simulink model "KALMAN_2D_test3"  (R2020a)
settings: Solver=VariableStepAuto  StartTime=0.0  StopTime=10  RelTol=1e-3
undefined symbols (not defined in the file): sigbuilder_block
libraries: simulink x3
settings Model: Creator=abdou  LastModifiedBy=abdou

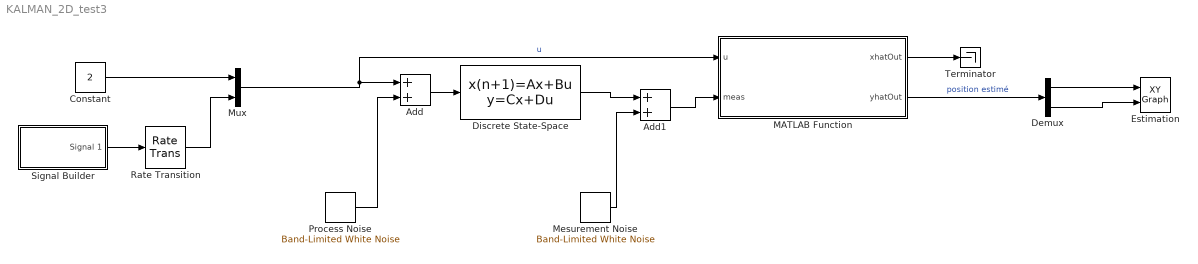
== system KALMAN_2D_test3 ==
  Add : Sum
  Add1 : Sum
  Constant : Constant  Value=2
  Demux : Demux  Outputs=2
  Discrete State-Space : DiscreteStateSpace  A=[1 0; 0 1]  B=[0.1 0; 0 0.1]  C=[1 0; 0 1]  D=[0 0; 0 0]  SampleTime=-1
  Estimation : simulink/Sinks/XY Graph  xmin=0  xmax=20  ymin=-0.2  ymax=0.2  st=-1
  MATLAB Function : MATLAB Function  TreatAsAtomicUnit=on
  Mesurement Noise : simulink/Sources/Band-Limited White Noise  Cov=[1 1]  Ts=0.1  seed=[23341]
  Mux : Mux  Inputs=2
  "Process Noise " : simulink/Sources/Band-Limited White Noise  Cov=[0.3 0.3]  Ts=0.1  seed=[23341]
  Rate Transition : RateTransition
  Signal Builder : Subsystem  Tag=STV Subsys  LoadFcn=sigbuilder_block('load');  StartFcn=sigbuilder_block('start');  StopFcn=sigbuilder_block('stop');  ClipboardFcn=sigbuilder_block('clipboard');  mask(Sigbuilder block){tuvar=[0:10]}
      mask help: Simulink:masks:SigbuilderBlock_MD
      mask init:
      | if ~strcmp(get_param(bdroot(gcbh),'SimulationStatus'),'stopped') tuvar = sigbuilder_block('maskInit'); end
      settings: CopyFcn=sigbuilder_block('copy');  DeleteFcn=sigbuilder_block('delete');  ModelCloseFcn=sigbuilder_block('modelClose');  PreSaveFcn=sigbuilder_block('preSave');  PauseFcn=sigbuilder_block('pause');  ContinueFcn=sigbuilder_block('continue');  NameChangeFcn=sigbuilder_block('namechange');  OpenFcn=sigbuilder_block('open',[6 30 1012.5 447.75 ]);  CloseFcn=sigbuilder_block('close');
      mask Display: plot(0, 0, 100, 100,[2, 2, 32, 32, 2], [68, 8, 8, 68, 68],[32, 2], [38, 38], [32, 19, 2],[53, 60, 44], [32, 17, 17, 2],[16, 16, 31, 31]);txt = getActiveGroup(gcbh);text(2, 100, txt,'verticalAlignment', 'top');
  Terminator : Terminator
  wires:
  Signal Builder/1(Signal 1) -> Rate Transition/1
  Rate Transition/1 -> Mux/2
  "Process Noise "/1 -> Add/2
  Add1/1 -> MATLAB Function/2(meas)
  Mesurement Noise/1 -> Add1/2
  Demux/1 -> Estimation/1
  Demux/2 -> Estimation/2
  Discrete State-Space/1 -> Add1/1
  Add/1 -> Discrete State-Space/1
  Constant/1 -> Mux/1
  MATLAB Function/2(yhatOut) -> Demux/1  "position estimé"
  Mux/1 -> MATLAB Function/1(u), Add/1  "u"
  MATLAB Function/1(xhatOut) -> Terminator/1

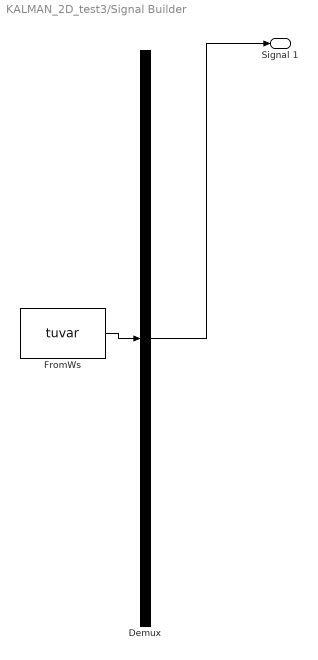
== system KALMAN_2D_test3/Signal Builder ==
  Demux : Demux  Tag=STV Demux  Outputs=1
      settings: DisplayOption=none
  FromWs : FromWorkspace  Tag=STV FromWs  VariableName=tuvar
      SigBuilderData=|
      | common.afterFinalStr = 'Extrapolate'
      | common.sampleTime = 0
      | dataSet.timeRange = [0 10]
      | dataSet.name = 'Group 1'
      | sbobj.Groups.Name = 'Group 1'
      | sbobj.Groups.Signals.Name = 'Signal 1'
      | sbobj.Groups.Signals.XData = [0 5.01 5.01 8 8 10]
      | sbobj.Groups.Signals.YData = [0 0 -1 0.99 -0.01 -0.01]
  Signal 1 : Outport  Tag=STV Outport
  wires:
  FromWs/1 -> Demux/1
  Demux/1 -> Signal 1/1

== matlab function KALMAN_2D_test3/MATLAB Function ==
  settings: updateMethod=DISCRETE
  data: u input; xhatOut output; meas input; yhatOut output
function [xhatOut, yhatOut] = KALMAN(u,meas)

% First time through the code so do some initialization
persistent P xhat A B C Q R
if isempty(P)
   xhat = [0 0]';
   A=[1 0; 0 0]; %define the state matrix
   C=[1 0; 0 1]; %define the output matrix
   B=[0.1 0; 0 0.1]; 
  %define the input matrixl
 
    %standard deviation ax
   segmaux = 7   ;
   segmaualpha= 7; %standard deviation angular speed
  
   measurmentsV=[250.^2  0  ; 0 300.^2];
   R=measurmentsV*C*(C');
   Q=[segmaux.^2 0 ;0 segmaualpha.^2];
   P= [0 0; 0 0];
end
% Propagate the state estimate and covariance matrix:
xhat = A*xhat + B*u;
P = A*P*A' + Q;
% Calculate the Kalman gain
K = P*C'/(C*P*C' + R);
% Calculate the measurement residual
resid = meas - C*xhat;
% Update the state and error covariance estimate
xhat = xhat + K*resid;
P = (eye(size(K,1))-K*C)*P;
% Post the results
xhatOut = xhat;
yhatOut = C*xhatOut;
